simulink model "Impedance_Control"  (R2021b)
settings: Solver=VariableStepAuto  StartTime=0.0  StopTime=10  RelTol=1e-3
undefined symbols (not defined in the file or in its folder): Dm, Km, q_dq_init
(part 1 of 3)
settings Model: Creator=ouyaf  LastModifiedBy=ouyaf

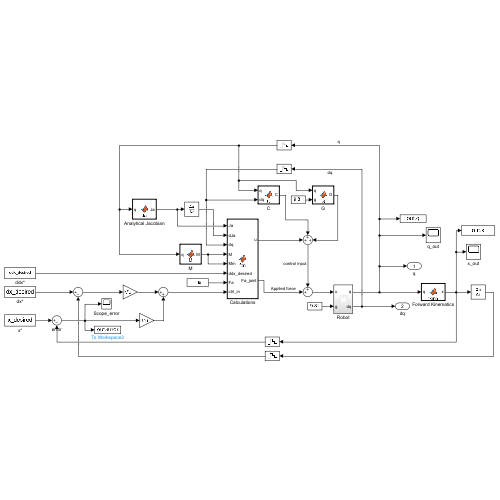
[thumbnail: Simulink's stored preview of the top-level diagram]
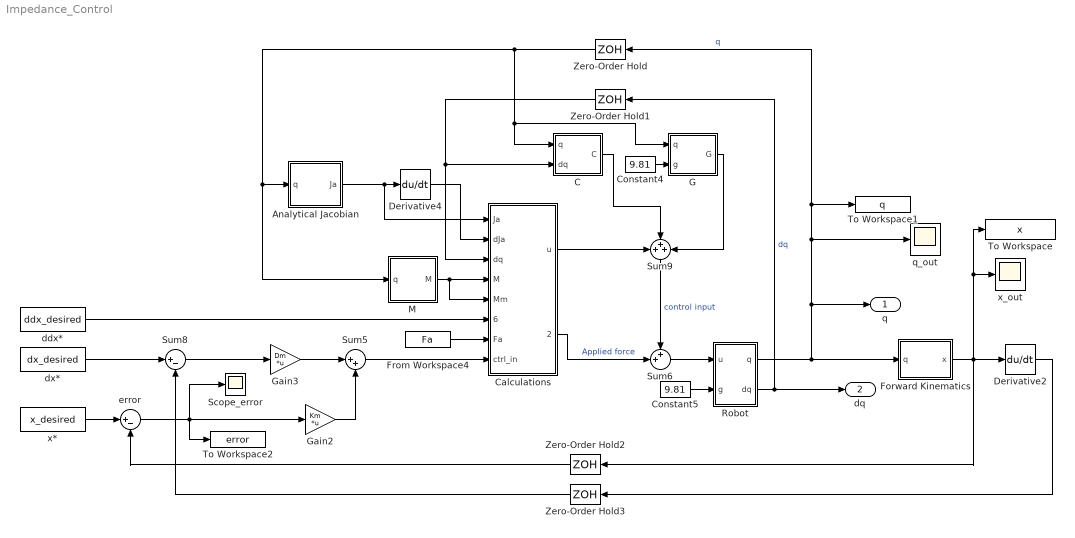
== system Impedance_Control ==
  Analytical Jacobian : MATLAB Function  TreatAsAtomicUnit=on
  C : MATLAB Function  TreatAsAtomicUnit=on
  Calculations : MATLAB Function  TreatAsAtomicUnit=on
  Constant4 : Constant  Value=9.81
  Constant5 : Constant  Value=9.81
  Derivative2 : Derivative
  Derivative4 : Derivative
  Forward Kinematics : MATLAB Function  TreatAsAtomicUnit=on
  From Workspace4 : FromWorkspace  VariableName=Fa
  G : MATLAB Function  TreatAsAtomicUnit=on
  Gain2 : Gain  Gain=Km  Multiplication=Matrix(K*u)
  Gain3 : Gain  Gain=Dm  Multiplication=Matrix(K*u)
  M : MATLAB Function  TreatAsAtomicUnit=on
  Robot : Subsystem
  Scope_error : Scope
  Sum5 : Sum  Inputs=|++
  Sum6 : Sum  Inputs=++|
  Sum8 : Sum  Inputs=|+-
  Sum9 : Sum  Inputs=+++
  To Workspace : ToWorkspace  VariableName=x  SaveFormat=Timeseries  SampleTime=-1
  To Workspace1 : ToWorkspace  VariableName=q  SaveFormat=Timeseries  SampleTime=-1
  To Workspace2 : ToWorkspace  VariableName=error  SaveFormat=Timeseries  SampleTime=-1
  Zero-Order Hold{,1..3} (4 alike) : ZeroOrderHold  SampleTime=0.001
  ddx* : FromWorkspace  VariableName=ddx_desired
  dx* : FromWorkspace  VariableName=dx_desired
  error : Sum  Inputs=|+-
  q_out : Scope
  x* : FromWorkspace  VariableName=x_desired
  x_out : Scope
  q : Outport  PortDimensions=6
  dq : Outport  Port=2  PortDimensions=6
  wires:
  Robot/2(dq) -> Zero-Order Hold1/1, dq/1  "dq"
  Constant4/1 -> G/2(g)
  Gain2/1 -> Sum5/2
  error/1 -> To Workspace2/1, Gain2/1, Scope_error/1
  G/1(G) -> Sum9/3
  Gain3/1 -> Sum5/1
  C/1(C) -> Sum9/2
  Sum8/1 -> Gain3/1
  Sum5/1 -> Calculations/8(ctrl_in)
  Calculations/1(u) -> Sum9/1
  Forward Kinematics/1(x) -> x_out/1, To Workspace/1, Zero-Order Hold2/1, Derivative2/1
  dx*/1 -> Sum8/1
  Derivative2/1 -> Zero-Order Hold3/1
  x*/1 -> error/1
  Analytical Jacobian/1(Ja) -> Calculations/1(Ja), Derivative4/1
  Derivative4/1 -> Calculations/2(dJa)
  From Workspace4/1 -> Calculations/7(Fa)
  M/1(M) -> Calculations/5(Mm), Calculations/4(M)
  ddx*/1 -> Calculations/6(ddx_desired)
  Sum9/1 -> Sum6/1  "control input"
  Calculations/2(Fa_joint) -> Sum6/2  "Applied force"
  Sum6/1 -> Robot/1(u)
  Constant5/1 -> Robot/2(g)
  Robot/1(q) -> Forward Kinematics/1(q), q/1, To Workspace1/1, Zero-Order Hold/1, q_out/1  "q"
  Zero-Order Hold/1 -> G/1(q), C/1(q), M/1(q), Analytical Jacobian/1(q)
  Zero-Order Hold1/1 -> C/2(dq), Calculations/3(dq)
  Zero-Order Hold2/1 -> error/2
  Zero-Order Hold3/1 -> Sum8/2

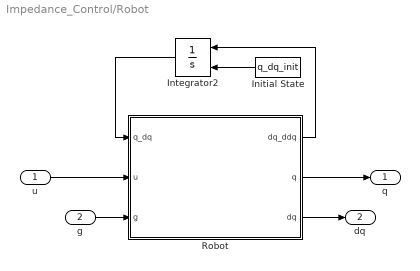
== system Impedance_Control/Robot ==
  u : Inport
  g : Inport  Port=2
  Initial State : Constant  Value=q_dq_init
  Integrator2 : Integrator  InitialConditionSource=external
  Robot : MATLAB Function  TreatAsAtomicUnit=on
  q : Outport
  dq : Outport  Port=2
  wires:
  Initial State/1 -> Integrator2/2
  Integrator2/1 -> Robot/1(q_dq)
  Robot/3(dq) -> dq/1
  Robot/1(dq_ddq) -> Integrator2/1
  g/1 -> Robot/3(g)
  u/1 -> Robot/2(u)
  Robot/2(q) -> q/1

== matlab function Impedance_Control/Calculations ==
  data: Ja input; u output; dJa input; dq input; M input; Mm input; ddx_desired input; Fa input; ctrl_in input; Fa_joint output
function [u,Fa_joint] = fcn(Ja, dJa, dq, M, Mm, ddx_desired, Fa, ctrl_in)

Mx = inv(Ja).'*M*inv(Ja);
Mm = Mx;

u = M/Ja*(ddx_desired - dJa*dq + Mm\(ctrl_in)) + Ja.'*(Mx/Mm - eye(6))*Fa;
% u = M*inv(Ja)*(ddx_desired - dJa*dq + inv(Mm)*(ctrl_in));
Fa_joint = Ja.'*Fa;
